simulink model "EfficiencySensitivityAnalysis"  (R2024b)
settings: Solver=FixedStepAuto  StartTime=0.0  StopTime=451.4  FixedStep=0.1  RelTol=1e-3
values from neighbouring files (symbols this model uses):
  GR = 6    [EfficiencySensitivityAnalysisParameters.m]
  mu_gb = 0.95    [EfficiencySensitivityAnalysisParameters.m]
  phi = 0    [EfficiencySensitivityAnalysisParameters.m]
  Tinit = 40    [EfficiencySensitivityAnalysisParameters.m]
  Tr = 0.33    [EfficiencySensitivityAnalysisParameters.m]
(part 1 of 3)
settings Model: Creator=rahulchakravarthula  LastModifiedBy=rahulchakravarthula

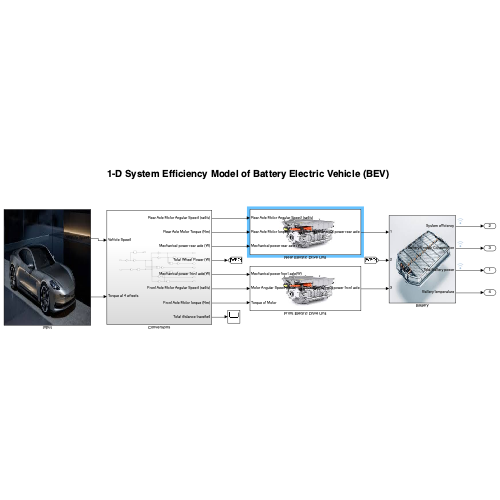
[thumbnail: Simulink's stored preview of the top-level diagram]
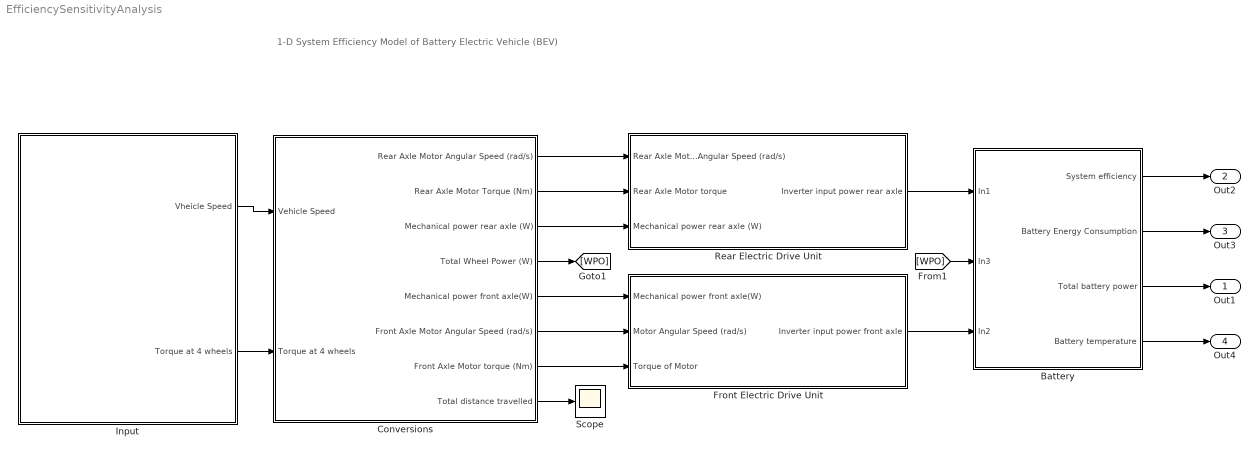
== system EfficiencySensitivityAnalysis ==
  note: 1-D System Efficiency Model of Battery Electric Vehicle (BEV)
  Battery : Subsystem
      mask Display: image('Unknown222.jpeg');
  Conversions : Subsystem
  Front Electric Drive Unit : Subsystem
      mask Display: image('Unknown.jpeg');
  Input : Subsystem
      mask Display: image('images.jpeg');
  Rear Electric Drive Unit : Subsystem
      mask Display: image('Unknown.jpeg');
  Scope : Scope
  Out1 : Outport
  Out2 : Outport  Port=2
  Out3 : Outport  Port=3
  Out4 : Outport  Port=4
  wires:
  Conversions/4(Total Wheel Power (W)) -> [WPO]
  Input/1(Vheicle Speed) -> Conversions/1(Vehicle Speed)
  Input/2(Torque at 4 wheels) -> Conversions/2(Torque at 4 wheels)
  Conversions/5(Mechanical power front axle(W)) -> Front Electric Drive Unit/1(Mechanical power front axle(W))
  Conversions/6(Front Axle Motor Angular Speed (rad/s)) -> Front Electric Drive Unit/2(Motor Angular Speed (rad/s))
  Conversions/7(" Front Axle Motor torque (Nm)") -> Front Electric Drive Unit/3(Torque of Motor)
  Conversions/1(Rear Axle Motor Angular Speed (rad/s)) -> Rear Electric Drive Unit/1(Rear Axle Motor Angular Speed (rad/s))
  Conversions/2(Rear Axle Motor Torque (Nm)) -> Rear Electric Drive Unit/2(Rear Axle Motor torque)
  Conversions/3(Mechanical power rear axle (W)) -> Rear Electric Drive Unit/3(Mechanical power rear axle (W))
  Rear Electric Drive Unit/1(Inverter input power rear axle) -> Battery/1(In1)
  Front Electric Drive Unit/1(Inverter input power front axle) -> Battery/3(In2)
  Battery/1(System efficiency) -> Out2/1
  Battery/2(Battery Energy Consumption) -> Out3/1
  Battery/3(Total battery power) -> Out1/1
  [WPO] -> Battery/2(In3)
  Conversions/8(Total distance travelled) -> Scope/1
  Battery/4(Battery temperature) -> Out4/1

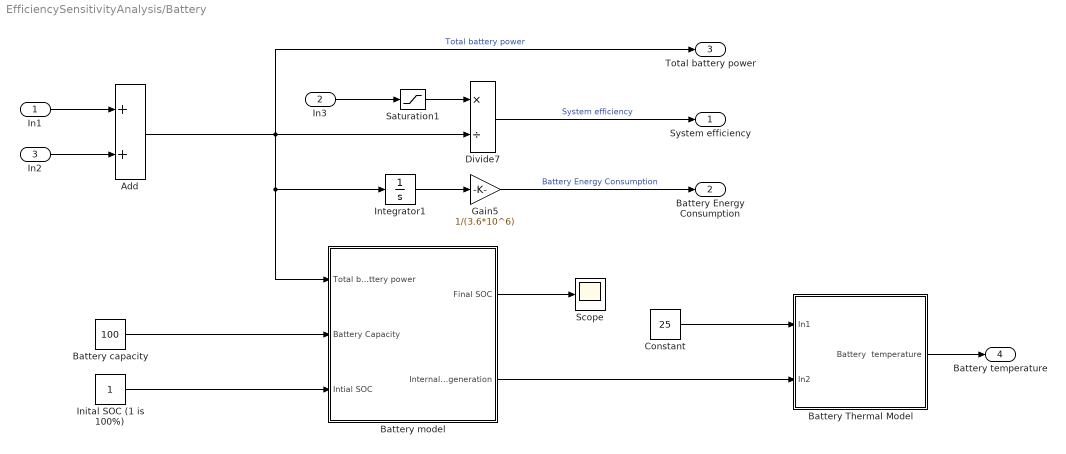
== system EfficiencySensitivityAnalysis/Battery ==
  In1 : Inport
  In3 : Inport  Port=2
  In2 : Inport  Port=3
  Add : Sum
  Battery Thermal Model : Subsystem
  Battery capacity : Constant  Value=100
  Battery model : Subsystem
  Constant : Constant  Value=25
  Divide7 : Product  Inputs=*/
  Gain5 : Gain  Gain=1/(3.6*10^6)
  Inital SOC (1 is 100%) : Constant
  Integrator1 : Integrator
  Saturation1 : Saturate  UpperLimit=10^6  LowerLimit=-3*10^6
  Scope : Scope
  System efficiency : Outport
  Battery Energy Consumption : Outport  Port=2
  Total battery power : Outport  Port=3
  Battery temperature : Outport  Port=4
  wires:
  In2/1 -> Add/2
  In1/1 -> Add/1
  Divide7/1 -> System efficiency/1  "System efficiency"
  Saturation1/1 -> Divide7/1
  Add/1 -> Total battery power/1, Divide7/2, Integrator1/1, Battery model/1(Total battery power)  "Total battery power"
  Gain5/1 -> Battery Energy Consumption/1  "Battery Energy Consumption"
  Integrator1/1 -> Gain5/1
  In3/1 -> Saturation1/1
  Battery capacity/1 -> Battery model/2(Battery Capacity)
  Inital SOC (1 is 100%)/1 -> Battery model/3(Intial SOC)
  Battery model/1(Final SOC) -> Scope/1
  Constant/1 -> Battery Thermal Model/1(In1)
  Battery model/2(Internal Heat generation) -> Battery Thermal Model/2(In2)
  Battery Thermal Model/1(Battery  temperature) -> Battery temperature/1

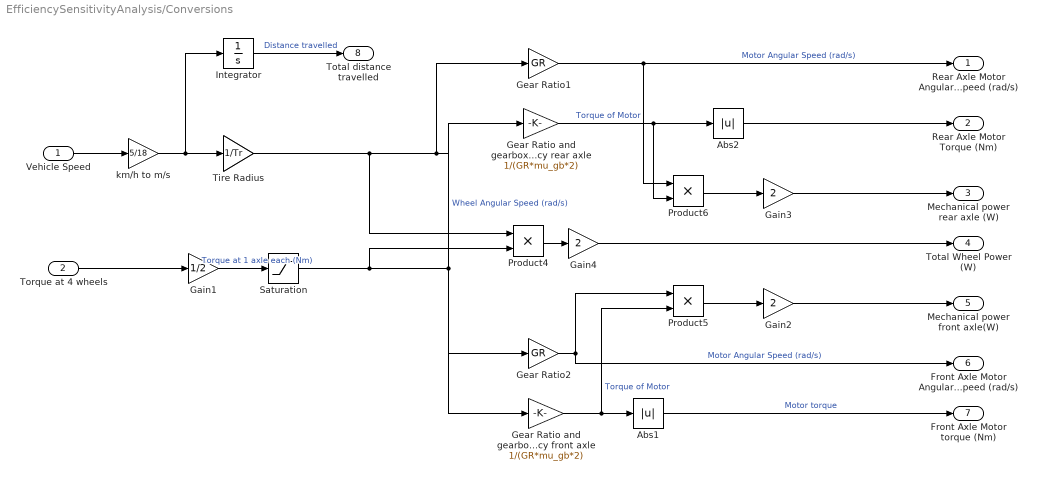
== system EfficiencySensitivityAnalysis/Conversions ==
  Vehicle Speed : Inport
  Torque at 4 wheels : Inport  Port=2
  Abs1 : Abs  SaturateOnIntegerOverflow=off
  Abs2 : Abs  SaturateOnIntegerOverflow=off
  Gain1 : Gain  Gain=1/2
  Gain2 : Gain  Gain=2
  Gain3 : Gain  Gain=2
  Gain4 : Gain  Gain=2
  Gear Ratio and gearbox efficiency front axle : Gain  Gain=1/(GR*mu_gb*2)
  Gear Ratio and gearbox efficiency rear axle : Gain  Gain=1/(GR*mu_gb*2)
  Gear Ratio1 : Gain  Gain=GR
  Gear Ratio2 : Gain  Gain=GR
  Integrator : Integrator
  Product4 : Product
  Product5 : Product
  Product6 : Product
  Saturation : Saturate  UpperLimit=4000  LowerLimit=-1000
  Tire Radius : Gain  Gain=1/Tr
  km/h to m/s : Gain  Gain=5/18
  Rear Axle Motor Angular Speed (rad/s) : Outport
  Rear Axle Motor Torque (Nm) : Outport  Port=2
  Mechanical power rear axle (W) : Outport  Port=3
  Total Wheel Power (W) : Outport  Port=4
  Mechanical power front axle(W) : Outport  Port=5
  Front Axle Motor Angular Speed (rad/s) : Outport  Port=6
  " Front Axle Motor torque (Nm)" : Outport  Port=7
  Total distance travelled : Outport  Port=8
  wires:
  Gain4/1 -> Total Wheel Power (W)/1
  Torque at 4 wheels/1 -> Gain1/1
  Abs1/1 -> " Front Axle Motor torque (Nm)"/1  "Motor torque"
  Vehicle Speed/1 -> km/h to m/s/1
  Gear Ratio1/1 -> Rear Axle Motor Angular Speed (rad/s)/1, Product6/1  "Motor Angular Speed (rad/s)"
  Gear Ratio and gearbox efficiency front axle/1 -> Product5/2, Abs1/1  "Torque of Motor"
  Tire Radius/1 -> Gear Ratio1/1, Gear Ratio2/1, Product4/1  "Wheel Angular Speed (rad/s)"
  Product4/1 -> Gain4/1
  Gain2/1 -> Mechanical power front axle(W)/1
  Gear Ratio and gearbox efficiency rear axle/1 -> Abs2/1, Product6/2  "Torque of Motor"
  Product6/1 -> Gain3/1
  Gain3/1 -> Mechanical power rear axle (W)/1
  Abs2/1 -> Rear Axle Motor Torque (Nm)/1
  km/h to m/s/1 -> Integrator/1, Tire Radius/1
  Gear Ratio2/1 -> Front Axle Motor Angular Speed (rad/s)/1, Product5/1  "Motor Angular Speed (rad/s)"
  Product5/1 -> Gain2/1
  Gain1/1 -> Saturation/1  "Torque at 1 axle each (Nm)"
  Integrator/1 -> Total distance travelled/1  "Distance travelled"
  Saturation/1 -> Gear Ratio and gearbox efficiency rear axle/1, Gear Ratio and gearbox efficiency front axle/1, Product4/2

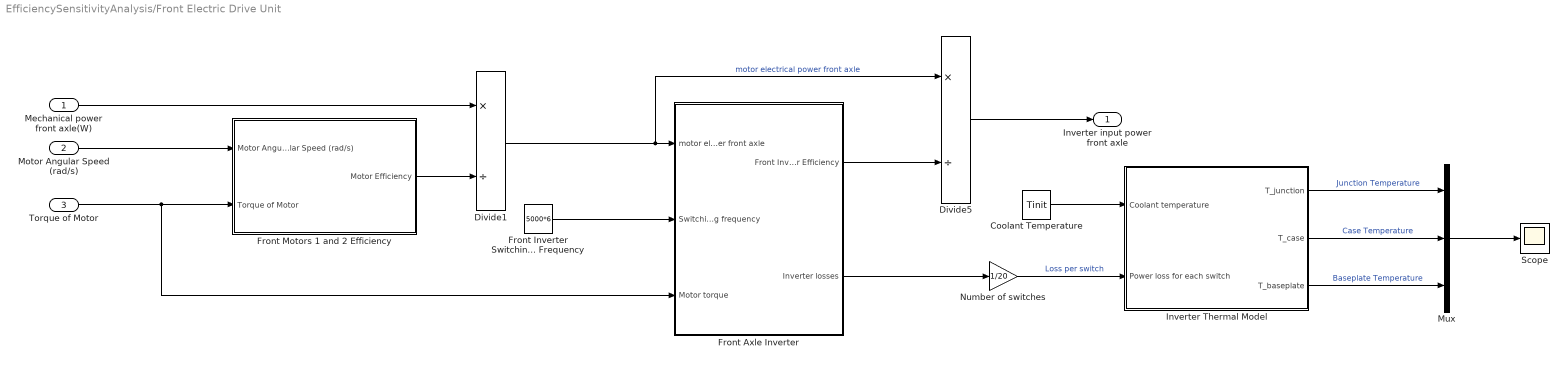
== system EfficiencySensitivityAnalysis/Front Electric Drive Unit ==
  Mechanical power front axle(W) : Inport
  Motor Angular Speed (rad/s) : Inport  Port=2
  Torque of Motor : Inport  Port=3
  Coolant Temperature : Constant  Value=Tinit
  Divide1 : Product  Inputs=*/
  Divide5 : Product  Inputs=*/
  Front Axle Inverter : Subsystem
  Front Inverter Switching Frequency : Constant  Value=5000*6
  "Front Motors 1 and 2 Efficiency " : Subsystem
  Inverter Thermal Model : Subsystem
  Mux : Mux  Inputs=3
  Number of switches : Gain  Gain=1/20
  Scope : Scope
  Inverter input power front axle : Outport
  wires:
  Motor Angular Speed (rad/s)/1 -> "Front Motors 1 and 2 Efficiency "/1(Motor Angular Speed (rad/s))
  Divide5/1 -> Inverter input power front axle/1
  "Front Motors 1 and 2 Efficiency "/1(Motor Efficiency) -> Divide1/2
  Front Axle Inverter/2(Inverter losses) -> Number of switches/1
  Front Inverter Switching Frequency/1 -> Front Axle Inverter/2(Switching frequency)
  Divide1/1 -> Front Axle Inverter/1(motor electrical power front axle), Divide5/1  "motor electrical power front axle"
  Torque of Motor/1 -> "Front Motors 1 and 2 Efficiency "/2(Torque of Motor), Front Axle Inverter/3(Motor torque)
  Front Axle Inverter/1(Front Inverter Efficiency) -> Divide5/2
  Mechanical power front axle(W)/1 -> Divide1/1
  Mux/1 -> Scope/1
  Inverter Thermal Model/2(T_case) -> Mux/2  "Case Temperature"
  Inverter Thermal Model/3(T_baseplate) -> Mux/3  "Baseplate Temperature"
  Coolant Temperature/1 -> Inverter Thermal Model/1(Coolant temperature)
  Number of switches/1 -> Inverter Thermal Model/2(Power loss for each switch)  "Loss per switch"
  Inverter Thermal Model/1(T_junction) -> Mux/1  "Junction Temperature"
